simulink model "es_motore_no_controllo_posiz"  (Simulink 8.3)
settings: Solver=ode45  StartTime=0.0  StopTime=20  RelTol=1e-6
values from neighbouring files (symbols this model uses):
  F1 = Ka*Km/((s*La+Ra)*(s*J+b)+Km^2)    [ES4_2.m]
  F2 = -(s*La+Ra)/((s*La+Ra)*(s*J+b)+Km^2)    [ES4_2.m]
  s = tf('s')    [ES4_2.m]
  Td_amp = 0.05    [ES4_2.m]
libraries: cstblocks x2
settings Model: Creator=Taragna  LastModifiedBy=Taragna  ExtModeTrigMode=oneshot  ExtModeArmWhenConnect=off
settings DataIOCC: LimitDataPoints=off
settings OptimizationCC: BlockReduction=off  BooleanDataType=off
settings DebuggingCC: SaveWithParameterizedLinksMsg=none  SignalResolutionControl=TryResolveAllWithWarning  SolverPrmCheckMsg=none  MultiTaskDSMMsg=warning  MultiTaskCondExecSysMsg=none  StateNameClashWarn=none  StrictBusMsg=None
settings HardwareCC: TargetUnknown=on
settings RTWCC: IncludeERTFirstTime=on

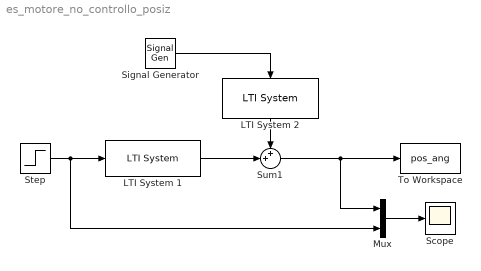
== system es_motore_no_controllo_posiz ==
  LTI System 1 : cstblocks/LTI System  sys=F1/s  IC=[0]
  LTI System 2 : cstblocks/LTI System  sys=F2/s  IC=[0]
  Mux : Mux  Inputs=2
  Scope : Scope
  Signal Generator : SignalGenerator  WaveForm=square  Amplitude=Td_amp  Frequency=0.1
  Step : Step  Time=0  SampleTime=0
  Sum1 : Sum  Inputs=++|  SaturateOnIntegerOverflow=on  InputSameDT=on  OutDataTypeStr=Inherit: Same as first input
  To Workspace : ToWorkspace  VariableName=pos_ang  SampleTime=-1
  wires:
  Mux/1 -> Scope/1
  LTI System 1/1 -> Sum1/2
  LTI System 2/1 -> Sum1/1
  Sum1/1 -> To Workspace/1, Mux/1
  Signal Generator/1 -> LTI System 2/1
  Step/1 -> LTI System 1/1, Mux/2
